simulink model "blocks_archive"  (R2019b)
settings: Solver=VariableStepAuto  StartTime=0.0  StopTime=10.0  RelTol=1e-3
values from neighbouring files (symbols this model uses):
  a = input("Semimajor axis [km]: ")    [SCARSSetup.m]    (also in pwsat2_setup.m = 6960989.91401; pwsat2_tle.m = 6960989.91401; scars_setup.m = 8000000; startup.m = 8000000)
  e = input("Eccentricity [-]: ")    [SCARSSetup.m]    (also in pwsat2_setup.m = 0.0011871; pwsat2_tle.m = 0.0011871; scars_setup.m = 0; startup.m = 0)
  G = 6.6743015e-11    [SCARSSetup.m]    (also in pwsat2_setup.m; pwsat2_tle.m; scars_setup.m; startup.m)
  h = norm(H)    [eci2kep.m]    (also in kep2eci.m = sqrt(a*mu*(1-e^2)); kep2rv.m = sqrt(a*mu*(1-e^2)); pwsat2_setup.m = 6378000; pwsat2_tle.m = 6378000)
  incl = input("Inclination [deg]: ")    [SCARSSetup.m]    (also in pwsat2_setup.m = deg2rad(97.7672); pwsat2_tle.m = deg2rad(97.7672); scars_setup.m = deg2rad(0.00000001); startup.m = deg2rad(45))
  Me = 5.972e24    (= 5.972e+24)    [SCARSSetup.m]    (also in pwsat2_setup.m; pwsat2_tle.m; scars_setup.m; startup.m)
  mu = 398600.4418    [eci2kep.m]    (also in pwsat2_setup.m = 398600441800000; pwsat2_tle.m = 398600441800000; scars_setup.m = 398600441800000; startup.m = 398600441800000)
  omega = 7.2921150e-5    (= 7.292115e-05)    [SCARSSetup.m]    (also in ec2ecef_test.m; pwsat2_setup.m; pwsat2_tle.m; scars_setup.m)
  RA = input("Right ascension of the ascending node [deg]: ")    [SCARSSetup.m]    (also in pwsat2_setup.m = deg2rad(56.1804); pwsat2_tle.m = deg2rad(56.1804); scars_setup.m = deg2rad(180); startup.m = deg2rad(90))
  TA = deg2rad(0)    [scars_setup.m]    (also in startup.m; startup_cubesat_ref.m = deg2rad(302.9234))
  v0 = [0 vy 0]    [startup.m]    (also in startup_cubesat_ref.m)
  w = input("Argument of periapsis [deg]: ")    [SCARSSetup.m]    (also in pwsat2_setup.m = deg2rad(236.0402); pwsat2_tle.m = deg2rad(236.0402); scars_setup.m = deg2rad(0); startup.m = deg2rad(0))
undefined symbols (not defined in the file or in its folder): IAU
libraries: sharedutil x6, aerolibgravity2 x2, aerolibtransform2 x1
settings Model: Creator=asmialek  LastModifiedBy=asmialek

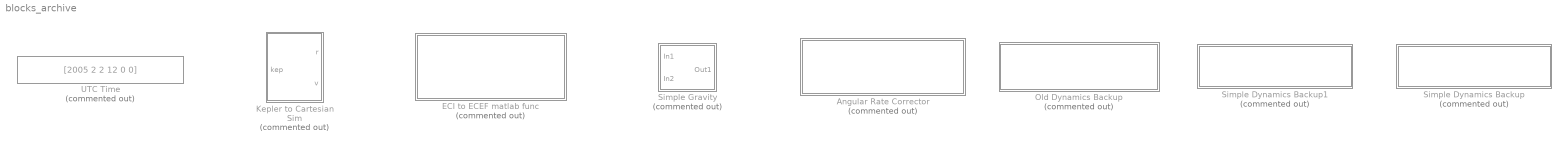
== system blocks_archive ==
  Angular Rate Corrector : Subsystem  Commented=on
  ECI to ECEF matlab func : Subsystem  Commented=on
  Kepler to Cartesian Sim : Subsystem  Commented=on
  Old Dynamics Backup : Subsystem  Commented=on
  Simple Dynamics Backup : Subsystem  Commented=on
  Simple Dynamics Backup1 : Subsystem  Commented=on
  Simple Gravity : Subsystem  Commented=on
  UTC Time : Constant  Commented=on  Value=[2005 2 2 12 0 0]

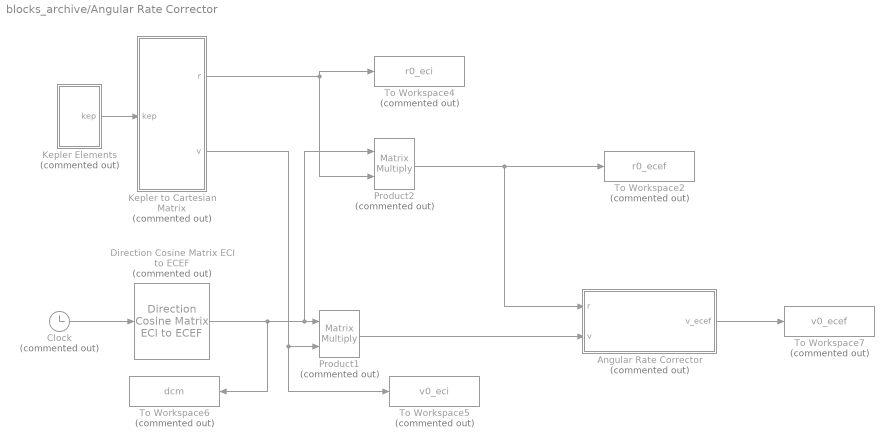
== system blocks_archive/Angular Rate Corrector ==
  Angular Rate Corrector : Subsystem  Commented=on
  Clock : Clock  Commented=on
  Direction Cosine Matrix ECI to ECEF : aerolibtransform2/Direction Cosine Matrix ECI to ECEF  Commented=on  red=IAU-2000/2006  year=2005  month=February  day=2  hour=12  min=0  sec=0  deltaT=Sec  errorflag=Error  extraparamflag=off
      settings: AttributesFormatString=%<red>  SourceProductName=Aerospace Blockset  SourceProductBaseCode=AE
  Kepler Elements : Subsystem  Commented=on
  Kepler to Cartesian Matrix : Subsystem  Commented=on
  Product1 : Product  Commented=on  Multiplication=Matrix(*)
  Product2 : Product  Commented=on  Multiplication=Matrix(*)
  To Workspace2 : ToWorkspace  Commented=on  VariableName=r0_ecef  SampleTime=-1
  To Workspace4 : ToWorkspace  Commented=on  VariableName=r0_eci  SampleTime=-1
  To Workspace5 : ToWorkspace  Commented=on  VariableName=v0_eci  SampleTime=-1
  To Workspace6 : ToWorkspace  Commented=on  VariableName=dcm  SampleTime=-1
  To Workspace7 : ToWorkspace  Commented=on  VariableName=v0_ecef  SampleTime=-1
  wires:
  Kepler to Cartesian Matrix/1(r) -> To Workspace4/1, Product2/2
  Direction Cosine Matrix ECI to ECEF/1 -> To Workspace6/1, Product2/1, Product1/1
  Clock/1 -> Direction Cosine Matrix ECI to ECEF/1
  Product1/1 -> Angular Rate Corrector/2(v)
  Product2/1 -> To Workspace2/1, Angular Rate Corrector/1(r)
  Kepler to Cartesian Matrix/2(v) -> To Workspace5/1, Product1/2
  Angular Rate Corrector/1(v_ecef) -> To Workspace7/1
  Kepler Elements/1(kep) -> Kepler to Cartesian Matrix/1(kep)

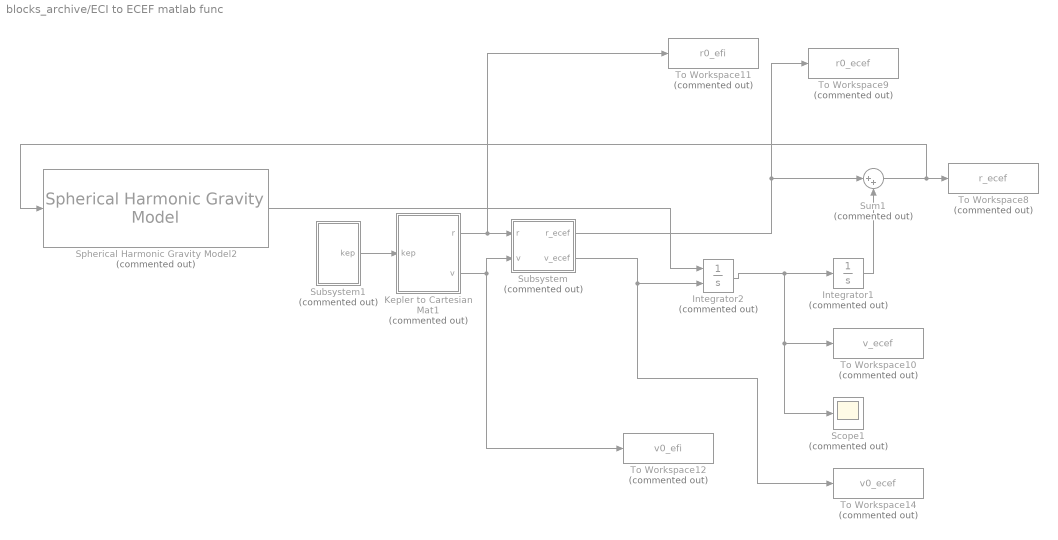
== system blocks_archive/ECI to ECEF matlab func ==
  Integrator1 : Integrator  Commented=on
  Integrator2 : Integrator  Commented=on  InitialConditionSource=external
  Kepler to Cartesian Mat1 : Subsystem  Commented=on
  Scope1 : Scope  Commented=on
  Spherical Harmonic Gravity Model2 : aerolibgravity2/Spherical Harmonic Gravity Model  Commented=on  units=Metric (MKS)  degree=120  action=Warning  ptype=EGM2008  datafile='aerogmm2b.mat'
      settings: SourceProductName=Aerospace Blockset  SourceProductBaseCode=AE
  Subsystem : Subsystem  Commented=on
  Subsystem1 : Subsystem  Commented=on
  Sum1 : Sum  Commented=on  Inputs=|++
  To Workspace10 : ToWorkspace  Commented=on  VariableName=v_ecef  SampleTime=-1
      settings: Save2DSignal=2-D array (concatenate along first dimension)
  To Workspace11 : ToWorkspace  Commented=on  VariableName=r0_efi  SampleTime=-1
  To Workspace12 : ToWorkspace  Commented=on  VariableName=v0_efi  SampleTime=-1
  To Workspace14 : ToWorkspace  Commented=on  VariableName=v0_ecef  SampleTime=-1
  To Workspace8 : ToWorkspace  Commented=on  VariableName=r_ecef  SampleTime=-1
  To Workspace9 : ToWorkspace  Commented=on  VariableName=r0_ecef  SampleTime=-1
  wires:
  Integrator2/1 -> Scope1/1, To Workspace10/1, Integrator1/1
  Sum1/1 -> To Workspace8/1, Spherical Harmonic Gravity Model2/1
  Kepler to Cartesian Mat1/2(v) -> Subsystem/2(v), To Workspace12/1
  Spherical Harmonic Gravity Model2/1 -> Integrator2/1
  Subsystem/1(r_ecef) -> To Workspace9/1, Sum1/1
  Integrator1/1 -> Sum1/2
  Subsystem1/1(kep) -> Kepler to Cartesian Mat1/1(kep)
  Kepler to Cartesian Mat1/1(r) -> To Workspace11/1, Subsystem/1(r)
  Subsystem/2(v_ecef) -> To Workspace14/1, Integrator2/2

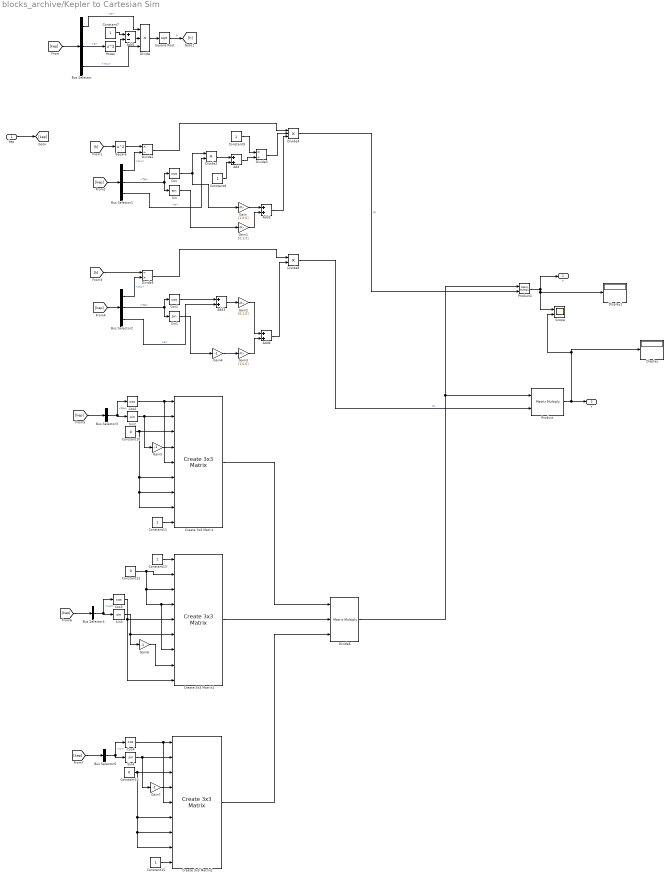
== system blocks_archive/Kepler to Cartesian Sim ==
  kep : Inport
  Add{,2..4} (4 alike) : Sum
  Add1 : Sum  Inputs=+-
  Bus Selector : BusSelector  OutputSignals=a,e,mu
  Bus Selector1 : BusSelector  OutputSignals=mu,TA,e
  Bus Selector2 : BusSelector  OutputSignals=mu,TA,e
  Bus Selector3 : BusSelector  OutputSignals=RA
  Bus Selector4 : BusSelector  OutputSignals=incl
  Bus Selector5 : BusSelector  OutputSignals=w
  Constant10 : Constant  Value=0
  Constant{7..9,11,13,15} (6 alike) : Constant
  Constant12 : Constant  Value=0
  Constant14 : Constant  Value=0
  Cos{,1..4} (5 alike) : Trigonometry  Operator=cos
  Create 3x3 Matrix : sharedutil/Create 3x3 Matrix  aMode=aMode
  Create 3x3 Matrix1 : sharedutil/Create 3x3 Matrix  aMode=aMode
  Create 3x3 Matrix2 : sharedutil/Create 3x3 Matrix  aMode=aMode
  Display : Display
  Display1 : Display
  Divide : Product  Inputs=3
  Divide1 : Product  Inputs=*/
  Divide2 : Product
  Divide3 : Product  Inputs=*/
  Divide4 : Product  Inputs=3
  Divide5 : Product  Inputs=/*
  Divide6 : Product  Inputs=3  Multiplication=Matrix(*)
  Divide8 : Product
  Gain : Gain  Gain=[1;0;0]
  Gain1 : Gain  Gain=[0;1;0]
  Gain2 : Gain  Gain=[0;1;0]
  Gain3 : Gain  Gain=[1;0;0]
  Gain{4..7} (4 alike) : Gain  Gain=-1
  Power : Math  Operator=square  SignedPower=off  SaturateOnIntegerOverflow=on
  Product : Product  Multiplication=Matrix(*)
  Product1 : Product  Multiplication=Matrix(*)
  Scope : Scope  NumInputPorts=2
  Sin{,1..4} (5 alike) : Trigonometry
  Square : Math  Operator=square  SignedPower=off  SaturateOnIntegerOverflow=on
  Square Root : Sqrt  SaturateOnIntegerOverflow=on
  r : Outport
  v : Outport  Port=2
  wires:
  Bus Selector2/1 -> Divide5/2  "<mu>"
  [h] -> Square/1
  Square Root/1 -> [h]  "h"
  Bus Selector2/3 -> Add3/2  "<e>"
  [kep] -> Bus Selector3/1
  Gain5/1 -> Create 3x3 Matrix/4
  Divide3/1 -> Divide4/2
  Constant15/1 -> Create 3x3 Matrix2/9
  Bus Selector1/1 -> Divide1/2  "<mu>"
  Gain6/1 -> Create 3x3 Matrix1/8
  Add/1 -> Divide3/2
  Create 3x3 Matrix2/1 -> Divide6/3
  Divide1/1 -> Divide4/1
  Sin1/1 -> Gain4/1
  Cos1/1 -> Add3/1
  Gain7/1 -> Create 3x3 Matrix2/4
  Gain3/1 -> Add4/2
  Cos2/1 -> Create 3x3 Matrix/5, Create 3x3 Matrix/1
  [kep] -> Bus Selector4/1
  Gain1/1 -> Add2/2
  Constant7/1 -> Add1/1
  Create 3x3 Matrix1/1 -> Divide6/2
  Divide5/1 -> Divide8/1
  Bus Selector4/1 -> Cos3/1, Sin3/1  "<incl>"
  Constant10/1 -> Create 3x3 Matrix/8, Create 3x3 Matrix/7, Create 3x3 Matrix/6, Create 3x3 Matrix/3
  Divide6/1 -> Product1/1, Product/1
  Cos3/1 -> Create 3x3 Matrix1/9, Create 3x3 Matrix1/5
  Power/1 -> Add1/2
  [kep] -> Bus Selector/1
  Constant12/1 -> Create 3x3 Matrix1/7, Create 3x3 Matrix1/4, Create 3x3 Matrix1/3, Create 3x3 Matrix1/2
  Bus Selector1/2 -> Cos/1, Sin/1  "<TA>"
  Bus Selector/3 -> Divide/3  "<mu>"
  Divide4/1 -> Product1/2  "rp"
  Bus Selector5/1 -> Cos4/1, Sin4/1  "<w>"
  Gain2/1 -> Add4/1
  Sin4/1 -> Gain7/1, Create 3x3 Matrix2/2
  Bus Selector1/3 -> Divide2/2  "<e>"
  [kep] -> Bus Selector5/1
  Gain4/1 -> Gain3/1
  Divide2/1 -> Add/1
  kep/1 -> [kep]
  [kep] -> Bus Selector1/1
  Sin3/1 -> Create 3x3 Matrix1/6, Gain6/1
  Divide8/1 -> Product/2  "vp"
  Constant13/1 -> Create 3x3 Matrix1/1
  [kep] -> Bus Selector2/1
  Bus Selector3/1 -> Cos2/1, Sin2/1  "<RA>"
  Constant8/1 -> Add/2
  Add4/1 -> Divide8/2
  Bus Selector/1 -> Divide/1  "<a>"
  Sin/1 -> Gain1/1
  Product1/1 -> r/1, Display1/1, Scope/1
  Bus Selector2/2 -> Cos1/1, Sin1/1  "<TA>"
  Add2/1 -> Divide4/3
  Add3/1 -> Gain2/1
  Constant11/1 -> Create 3x3 Matrix/9
  Constant14/1 -> Create 3x3 Matrix2/8, Create 3x3 Matrix2/7, Create 3x3 Matrix2/6, Create 3x3 Matrix2/3
  Create 3x3 Matrix/1 -> Divide6/1
  Product/1 -> v/1, Display/1, Scope/2
  Add1/1 -> Divide/2
  [h] -> Divide5/1
  Divide/1 -> Square Root/1
  Bus Selector/2 -> Power/1  "<e>"
  Cos4/1 -> Create 3x3 Matrix2/5, Create 3x3 Matrix2/1
  Sin2/1 -> Gain5/1, Create 3x3 Matrix/2
  Square/1 -> Divide1/1
  Cos/1 -> Divide2/1, Gain/1
  Constant9/1 -> Divide3/1
  Gain/1 -> Add2/1

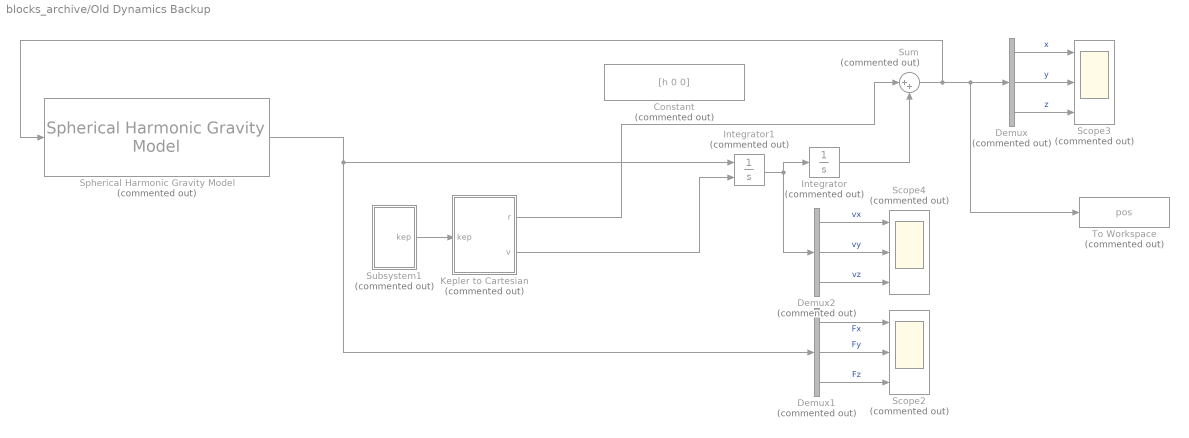
== system blocks_archive/Old Dynamics Backup ==
  Constant : Constant  Commented=on  Value=[h 0 0]
  Demux : Demux  Commented=on  Outputs=3
  Demux1 : Demux  Commented=on  Outputs=3
  Demux2 : Demux  Commented=on  Outputs=3
  Integrator : Integrator  Commented=on
  Integrator1 : Integrator  Commented=on  InitialConditionSource=external  InitialCondition=v0
  Kepler to Cartesian : Subsystem  Commented=on
  Scope2 : Scope  Commented=on  NumInputPorts=3
  Scope3 : Scope  Commented=on  NumInputPorts=3
  Scope4 : Scope  Commented=on  NumInputPorts=3
  Spherical Harmonic Gravity Model : aerolibgravity2/Spherical Harmonic Gravity Model  Commented=on  units=Metric (MKS)  degree=120  action=Warning  ptype=EGM2008  datafile='aerogmm2b.mat'
      settings: SourceProductName=Aerospace Blockset  SourceProductBaseCode=AE
  Subsystem1 : Subsystem  Commented=on
  Sum : Sum  Commented=on  Inputs=|++
  To Workspace : ToWorkspace  Commented=on  VariableName=pos  SampleTime=-1
  wires:
  Demux/1 -> Scope3/1  "x"
  Demux/3 -> Scope3/3  "z"
  Subsystem1/1(kep) -> Kepler to Cartesian/1(kep)
  Demux1/1 -> Scope2/1  "Fx"
  Kepler to Cartesian/2(v) -> Integrator1/2
  Demux1/2 -> Scope2/2  "Fy"
  Integrator1/1 -> Integrator/1, Demux2/1
  Demux1/3 -> Scope2/3  "Fz"
  Spherical Harmonic Gravity Model/1 -> Integrator1/1, Demux1/1
  Demux2/3 -> Scope4/3  "vz"
  Sum/1 -> To Workspace/1, Demux/1, Spherical Harmonic Gravity Model/1
  Kepler to Cartesian/1(r) -> Sum/1
  Demux2/2 -> Scope4/2  "vy"
  Integrator/1 -> Sum/2
  Demux/2 -> Scope3/2  "y"
  Demux2/1 -> Scope4/1  "vx"

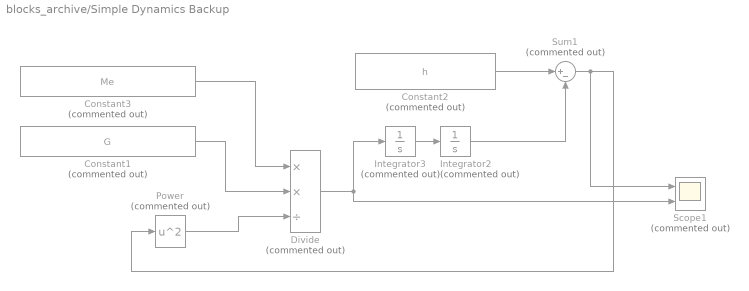
== system blocks_archive/Simple Dynamics Backup ==
  Constant1 : Constant  Commented=on  Value=G
  Constant2 : Constant  Commented=on  Value=h
  Constant3 : Constant  Commented=on  Value=Me
  Divide : Product  Commented=on  Inputs=**/
  Integrator2 : Integrator  Commented=on
  Integrator3 : Integrator  Commented=on
  Power : Math  Commented=on  Operator=square  SignedPower=off  SaturateOnIntegerOverflow=on
  Scope1 : Scope  Commented=on  NumInputPorts=2
  Sum1 : Sum  Commented=on  Inputs=|+-
  wires:
  Constant2/1 -> Sum1/1
  Constant1/1 -> Divide/2
  Integrator3/1 -> Integrator2/1
  Constant3/1 -> Divide/1
  Power/1 -> Divide/3
  Divide/1 -> Integrator3/1, Scope1/2
  Integrator2/1 -> Sum1/2
  Sum1/1 -> Scope1/1, Power/1

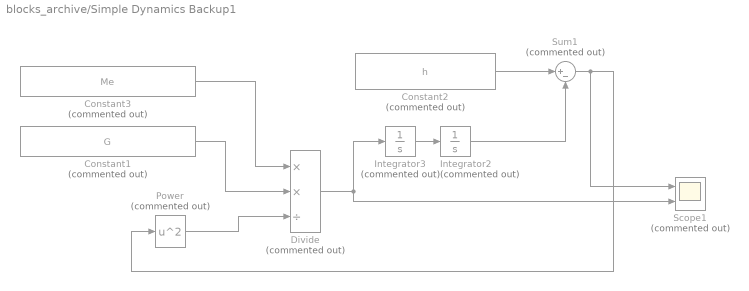
== system blocks_archive/Simple Dynamics Backup1 ==
  Constant1 : Constant  Commented=on  Value=G
  Constant2 : Constant  Commented=on  Value=h
  Constant3 : Constant  Commented=on  Value=Me
  Divide : Product  Commented=on  Inputs=**/
  Integrator2 : Integrator  Commented=on
  Integrator3 : Integrator  Commented=on
  Power : Math  Commented=on  Operator=square  SignedPower=off  SaturateOnIntegerOverflow=on
  Scope1 : Scope  Commented=on  NumInputPorts=2
  Sum1 : Sum  Commented=on  Inputs=|+-
  wires:
  Constant2/1 -> Sum1/1
  Constant1/1 -> Divide/2
  Integrator3/1 -> Integrator2/1
  Constant3/1 -> Divide/1
  Power/1 -> Divide/3
  Divide/1 -> Integrator3/1, Scope1/2
  Integrator2/1 -> Sum1/2
  Sum1/1 -> Scope1/1, Power/1

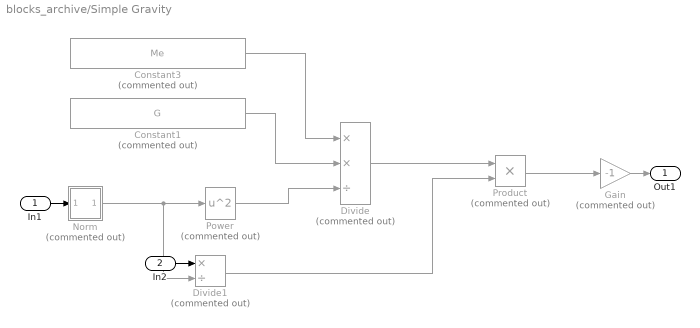
== system blocks_archive/Simple Gravity ==
  In1 : Inport
  In2 : Inport  Port=2
  Constant1 : Constant  Commented=on  Value=G
  Constant3 : Constant  Commented=on  Value=Me
  Divide : Product  Commented=on  Inputs=**/
  Divide1 : Product  Commented=on  Inputs=*/
  Gain : Gain  Commented=on  Gain=-1
  Norm : Subsystem  Commented=on
  Power : Math  Commented=on  Operator=square  SignedPower=off  SaturateOnIntegerOverflow=on
  Product : Product  Commented=on
  Out1 : Outport
  wires:
  Divide/1 -> Product/1
  Power/1 -> Divide/3
  Constant1/1 -> Divide/2
  In1/1 -> Norm/1(In1)
  Divide1/1 -> Product/2
  Norm/1(Out1) -> Divide1/2, Power/1
  Product/1 -> Gain/1
  Constant3/1 -> Divide/1
  Gain/1 -> Out1/1
  In2/1 -> Divide1/1

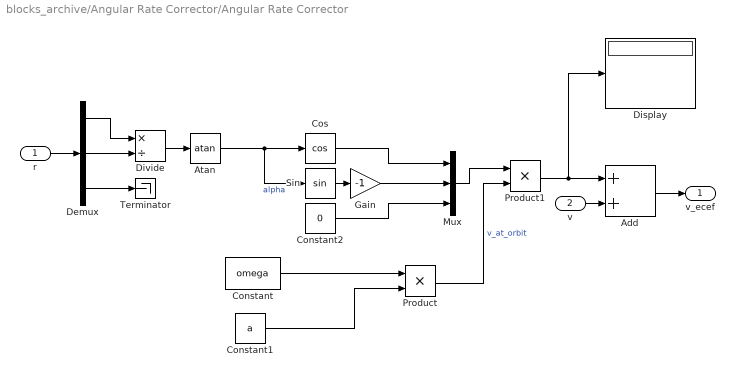
== system blocks_archive/Angular Rate Corrector/Angular Rate Corrector ==
  r : Inport
  v : Inport  Port=2
  Add : Sum
  Atan : Trigonometry  Operator=atan
  Constant : Constant  Value=omega
  Constant1 : Constant  Value=a
  Constant2 : Constant  Value=0
  Cos : Trigonometry  Operator=cos
  Demux : Demux  Outputs=3
  Display : Display
  Divide : Product  Inputs=*/
  Gain : Gain  Gain=-1
  Mux : Mux  Inputs=3
  Product : Product
  Product1 : Product
  Sin : Trigonometry
  Terminator : Terminator
  v_ecef : Outport
  wires:
  Add/1 -> v_ecef/1
  Product1/1 -> Display/1, Add/1
  r/1 -> Demux/1
  Demux/1 -> Divide/1
  Demux/2 -> Divide/2
  Divide/1 -> Atan/1
  Demux/3 -> Terminator/1
  Atan/1 -> Sin/1, Cos/1  "alpha"
  Constant/1 -> Product/1
  Constant1/1 -> Product/2
  Product/1 -> Product1/2  "v_at_orbit"
  v/1 -> Add/2
  Constant2/1 -> Mux/3
  Cos/1 -> Mux/1
  Sin/1 -> Gain/1
  Gain/1 -> Mux/2
  Mux/1 -> Product1/1

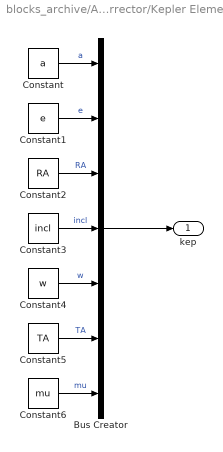
== system blocks_archive/Angular Rate Corrector/Kepler Elements ==
  Bus Creator : BusCreator  Inputs=7
  Constant : Constant  Value=a
  Constant1 : Constant  Value=e
  Constant2 : Constant  Value=RA
  Constant3 : Constant  Value=incl
  Constant4 : Constant  Value=w
  Constant5 : Constant  Value=TA
  Constant6 : Constant  Value=mu
  kep : Outport
  wires:
  Constant4/1 -> Bus Creator/5  "w"
  Constant/1 -> Bus Creator/1  "a"
  Bus Creator/1 -> kep/1
  Constant2/1 -> Bus Creator/3  "RA"
  Constant1/1 -> Bus Creator/2  "e"
  Constant3/1 -> Bus Creator/4  "incl"
  Constant5/1 -> Bus Creator/6  "TA"
  Constant6/1 -> Bus Creator/7  "mu"

== system blocks_archive/Angular Rate Corrector/Kepler to Cartesian Matrix ==
  kep : Inport
  Bus Selector : BusSelector  OutputSignals=a,e,RA,incl,w,TA,mu
  MATLAB Function : MATLAB Function  TreatAsAtomicUnit=on
  r : Outport
  v : Outport  Port=2
  wires:
  kep/1 -> Bus Selector/1
  Bus Selector/1 -> MATLAB Function/1(a)  "<a>"
  Bus Selector/2 -> MATLAB Function/2(e)  "<e>"
  Bus Selector/4 -> MATLAB Function/4(incl)  "<incl>"
  Bus Selector/5 -> MATLAB Function/5(w)  "<w>"
  Bus Selector/6 -> MATLAB Function/6(TA)  "<TA>"
  Bus Selector/7 -> MATLAB Function/7(mu)  "<mu>"
  Bus Selector/3 -> MATLAB Function/3(RA)  "<RA>"
  MATLAB Function/1(r) -> r/1
  MATLAB Function/2(v) -> v/1

== system blocks_archive/ECI to ECEF matlab func/Kepler to Cartesian Mat1 ==
  kep : Inport
  Bus Selector : BusSelector  OutputSignals=a,e,RA,incl,w,TA,mu
  MATLAB Function : MATLAB Function  TreatAsAtomicUnit=on
  r : Outport
  v : Outport  Port=2
  wires:
  kep/1 -> Bus Selector/1
  Bus Selector/1 -> MATLAB Function/1(a)  "<a>"
  Bus Selector/2 -> MATLAB Function/2(e)  "<e>"
  Bus Selector/4 -> MATLAB Function/4(incl)  "<incl>"
  Bus Selector/5 -> MATLAB Function/5(w)  "<w>"
  Bus Selector/6 -> MATLAB Function/6(TA)  "<TA>"
  Bus Selector/7 -> MATLAB Function/7(mu)  "<mu>"
  Bus Selector/3 -> MATLAB Function/3(RA)  "<RA>"
  MATLAB Function/1(r) -> r/1
  MATLAB Function/2(v) -> v/1

== system blocks_archive/ECI to ECEF matlab func/Subsystem ==
  r : Inport
  v : Inport  Port=2
  Constant : Constant  Value=[0 0 0]
  Constant1 : Constant  Value=2453404
  MATLAB Function : MATLAB Function  TreatAsAtomicUnit=on
  Terminator : Terminator
  r_ecef : Outport
  v_ecef : Outport  Port=2
  wires:
  Constant/1 -> MATLAB Function/4(a_ECI)
  v/1 -> MATLAB Function/3(v_ECI)
  MATLAB Function/2(v_ECEF) -> v_ecef/1
  MATLAB Function/3(a_ECEF) -> Terminator/1
  Constant1/1 -> MATLAB Function/1(JD)
  MATLAB Function/1(r_ECEF) -> r_ecef/1
  r/1 -> MATLAB Function/2(r_ECI)

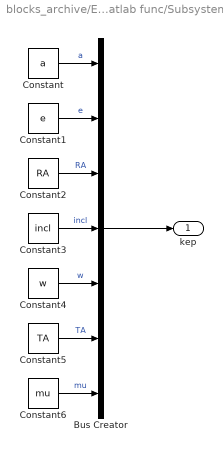
== system blocks_archive/ECI to ECEF matlab func/Subsystem1 ==
  Bus Creator : BusCreator  Inputs=7
  Constant : Constant  Value=a
  Constant1 : Constant  Value=e
  Constant2 : Constant  Value=RA
  Constant3 : Constant  Value=incl
  Constant4 : Constant  Value=w
  Constant5 : Constant  Value=TA
  Constant6 : Constant  Value=mu
  kep : Outport
  wires:
  Constant4/1 -> Bus Creator/5  "w"
  Constant/1 -> Bus Creator/1  "a"
  Bus Creator/1 -> kep/1
  Constant2/1 -> Bus Creator/3  "RA"
  Constant1/1 -> Bus Creator/2  "e"
  Constant3/1 -> Bus Creator/4  "incl"
  Constant5/1 -> Bus Creator/6  "TA"
  Constant6/1 -> Bus Creator/7  "mu"

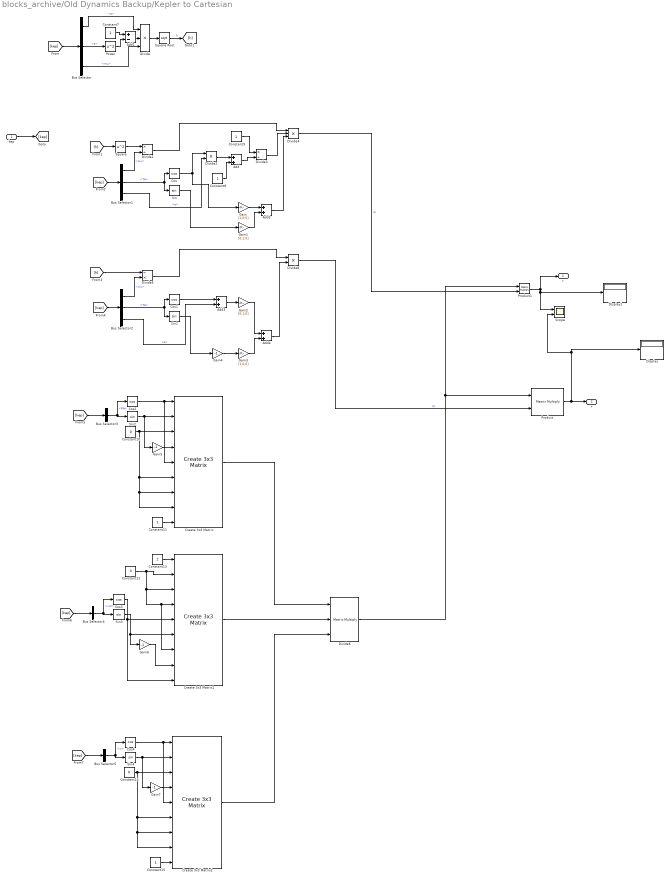
== system blocks_archive/Old Dynamics Backup/Kepler to Cartesian ==
  kep : Inport
  Add{,2..4} (4 alike) : Sum
  Add1 : Sum  Inputs=+-
  Bus Selector : BusSelector  OutputSignals=a,e,mu
  Bus Selector1 : BusSelector  OutputSignals=mu,TA,e
  Bus Selector2 : BusSelector  OutputSignals=mu,TA,e
  Bus Selector3 : BusSelector  OutputSignals=RA
  Bus Selector4 : BusSelector  OutputSignals=incl
  Bus Selector5 : BusSelector  OutputSignals=w
  Constant10 : Constant  Value=0
  Constant{7..9,11,13,15} (6 alike) : Constant
  Constant12 : Constant  Value=0
  Constant14 : Constant  Value=0
  Cos{,1..4} (5 alike) : Trigonometry  Operator=cos
  Create 3x3 Matrix : sharedutil/Create 3x3 Matrix  aMode=aMode
  Create 3x3 Matrix1 : sharedutil/Create 3x3 Matrix  aMode=aMode
  Create 3x3 Matrix2 : sharedutil/Create 3x3 Matrix  aMode=aMode
  Display : Display
  Display1 : Display
  Divide : Product  Inputs=3
  Divide1 : Product  Inputs=*/
  Divide2 : Product
  Divide3 : Product  Inputs=*/
  Divide4 : Product  Inputs=3
  Divide5 : Product  Inputs=/*
  Divide6 : Product  Inputs=3  Multiplication=Matrix(*)
  Divide8 : Product
  Gain : Gain  Gain=[1;0;0]
  Gain1 : Gain  Gain=[0;1;0]
  Gain2 : Gain  Gain=[0;1;0]
  Gain3 : Gain  Gain=[1;0;0]
  Gain{4..7} (4 alike) : Gain  Gain=-1
  Power : Math  Operator=square  SignedPower=off  SaturateOnIntegerOverflow=on
  Product : Product  Multiplication=Matrix(*)
  Product1 : Product  Multiplication=Matrix(*)
  Scope : Scope  NumInputPorts=2
  Sin{,1..4} (5 alike) : Trigonometry
  Square : Math  Operator=square  SignedPower=off  SaturateOnIntegerOverflow=on
  Square Root : Sqrt  SaturateOnIntegerOverflow=on
  r : Outport
  v : Outport  Port=2
  wires:
  Bus Selector2/1 -> Divide5/2  "<mu>"
  [h] -> Square/1
  Square Root/1 -> [h]  "h"
  Bus Selector2/3 -> Add3/2  "<e>"
  [kep] -> Bus Selector3/1
  Gain5/1 -> Create 3x3 Matrix/4
  Divide3/1 -> Divide4/2
  Constant15/1 -> Create 3x3 Matrix2/9
  Bus Selector1/1 -> Divide1/2  "<mu>"
  Gain6/1 -> Create 3x3 Matrix1/8
  Add/1 -> Divide3/2
  Create 3x3 Matrix2/1 -> Divide6/3
  Divide1/1 -> Divide4/1
  Sin1/1 -> Gain4/1
  Cos1/1 -> Add3/1
  Gain7/1 -> Create 3x3 Matrix2/4
  Gain3/1 -> Add4/2
  Cos2/1 -> Create 3x3 Matrix/5, Create 3x3 Matrix/1
  [kep] -> Bus Selector4/1
  Gain1/1 -> Add2/2
  Constant7/1 -> Add1/1
  Create 3x3 Matrix1/1 -> Divide6/2
  Divide5/1 -> Divide8/1
  Bus Selector4/1 -> Cos3/1, Sin3/1  "<incl>"
  Constant10/1 -> Create 3x3 Matrix/8, Create 3x3 Matrix/7, Create 3x3 Matrix/6, Create 3x3 Matrix/3
  Divide6/1 -> Product1/1, Product/1
  Cos3/1 -> Create 3x3 Matrix1/9, Create 3x3 Matrix1/5
  Power/1 -> Add1/2
  [kep] -> Bus Selector/1
  Constant12/1 -> Create 3x3 Matrix1/7, Create 3x3 Matrix1/4, Create 3x3 Matrix1/3, Create 3x3 Matrix1/2
  Bus Selector1/2 -> Cos/1, Sin/1  "<TA>"
  Bus Selector/3 -> Divide/3  "<mu>"
  Divide4/1 -> Product1/2  "rp"
  Bus Selector5/1 -> Cos4/1, Sin4/1  "<w>"
  Gain2/1 -> Add4/1
  Sin4/1 -> Gain7/1, Create 3x3 Matrix2/2
  Bus Selector1/3 -> Divide2/2  "<e>"
  [kep] -> Bus Selector5/1
  Gain4/1 -> Gain3/1
  Divide2/1 -> Add/1
  kep/1 -> [kep]
  [kep] -> Bus Selector1/1
  Sin3/1 -> Create 3x3 Matrix1/6, Gain6/1
  Divide8/1 -> Product/2  "vp"
  Constant13/1 -> Create 3x3 Matrix1/1
  [kep] -> Bus Selector2/1
  Bus Selector3/1 -> Cos2/1, Sin2/1  "<RA>"
  Constant8/1 -> Add/2
  Add4/1 -> Divide8/2
  Bus Selector/1 -> Divide/1  "<a>"
  Sin/1 -> Gain1/1
  Product1/1 -> r/1, Display1/1, Scope/1
  Bus Selector2/2 -> Cos1/1, Sin1/1  "<TA>"
  Add2/1 -> Divide4/3
  Add3/1 -> Gain2/1
  Constant11/1 -> Create 3x3 Matrix/9
  Constant14/1 -> Create 3x3 Matrix2/8, Create 3x3 Matrix2/7, Create 3x3 Matrix2/6, Create 3x3 Matrix2/3
  Create 3x3 Matrix/1 -> Divide6/1
  Product/1 -> v/1, Display/1, Scope/2
  Add1/1 -> Divide/2
  [h] -> Divide5/1
  Divide/1 -> Square Root/1
  Bus Selector/2 -> Power/1  "<e>"
  Cos4/1 -> Create 3x3 Matrix2/5, Create 3x3 Matrix2/1
  Sin2/1 -> Gain5/1, Create 3x3 Matrix/2
  Square/1 -> Divide1/1
  Cos/1 -> Divide2/1, Gain/1
  Constant9/1 -> Divide3/1
  Gain/1 -> Add2/1

== system blocks_archive/Old Dynamics Backup/Subsystem1 ==
  Bus Creator : BusCreator  Inputs=7
  Constant : Constant  Value=a
  Constant1 : Constant  Value=e
  Constant2 : Constant  Value=RA
  Constant3 : Constant  Value=incl
  Constant4 : Constant  Value=w
  Constant5 : Constant  Value=TA
  Constant6 : Constant  Value=mu
  kep : Outport
  wires:
  Constant4/1 -> Bus Creator/5  "w"
  Constant/1 -> Bus Creator/1  "a"
  Bus Creator/1 -> kep/1
  Constant2/1 -> Bus Creator/3  "RA"
  Constant1/1 -> Bus Creator/2  "e"
  Constant3/1 -> Bus Creator/4  "incl"
  Constant5/1 -> Bus Creator/6  "TA"
  Constant6/1 -> Bus Creator/7  "mu"

== system blocks_archive/Simple Gravity/Norm ==
  In1 : Inport
  Dot Product : DotProduct  InputSameDT=on  OutDataTypeStr=Inherit: Inherit via internal rule
  Square Root : Sqrt  SaturateOnIntegerOverflow=on
  Out1 : Outport
  wires:
  Dot Product/1 -> Square Root/1
  In1/1 -> Dot Product/2, Dot Product/1
  Square Root/1 -> Out1/1

== matlab function blocks_archive/ECI to ECEF matlab func/Kepler to Cartesian Mat1/MATLAB Function ==
  data: a input; r output; e input; RA input; incl input; w input; TA input; mu input; v output
% h - angular momentum (km^2/s)
% e - eccentricity (unitless)
% RA - right ascension of the ascending node (rad)
% incl - inclination (rad)
% w - argument of periapis (rad)
% TA - true anomaly (rad)
% mu - standard gravitational parameter (m^3/s^2)

function [r, v] = kep2rv(a, e, RA, incl, w, TA, mu)

h = sqrt(a*mu*(1-e^2));

rp = (h^2/mu) * (1/(1 + e.*cos(TA))) * (cos(TA).*[1;0;0] + sin(TA).*[0;1;0]);
vp = (mu/h) * (-sin(TA).*[1;0;0] + (e + cos(TA)).*[0;1;0]);

R3_W = [ cos(RA) sin(RA) 0;
         -sin(RA) cos(RA) 0;
         0          0       1];
     
R1_i = [1 0 0;
        0 cos(incl) sin(incl);
        0 -sin(incl) cos(incl)];
    
R3_w = [ cos(w) sin(w) 0;
         -sin(w) cos(w) 0;
         0 0 1];
     
Q_pX = (R3_w*R1_i*R3_W)';

r = Q_pX*rp;
v = Q_pX*vp;

r = r;
v = v;

end

== matlab function blocks_archive/Angular Rate Corrector/Kepler to Cartesian Matrix/MATLAB Function ==
  data: a input; r output; e input; RA input; incl input; w input; TA input; mu input; v output
% h - angular momentum (km^2/s)
% e - eccentricity (unitless)
% RA - right ascension of the ascending node (rad)
% incl - inclination (rad)
% w - argument of periapis (rad)
% TA - true anomaly (rad)
% mu - standard gravitational parameter (m^3/s^2)

function [r, v] = kep2rv(a, e, RA, incl, w, TA, mu)

h = sqrt(a*mu*(1-e^2));

rp = (h^2/mu) * (1/(1 + e.*cos(TA))) * (cos(TA).*[1;0;0] + sin(TA).*[0;1;0]);
vp = (mu/h) * (-sin(TA).*[1;0;0] + (e + cos(TA)).*[0;1;0]);

R3_W = [ cos(RA) sin(RA) 0;
         -sin(RA) cos(RA) 0;
         0          0       1];
     
R1_i = [1 0 0;
        0 cos(incl) sin(incl);
        0 -sin(incl) cos(incl)];
    
R3_w = [ cos(w) sin(w) 0;
         -sin(w) cos(w) 0;
         0 0 1];
     
Q_pX = (R3_w*R1_i*R3_W)';

r = Q_pX*rp;
v = Q_pX*vp;

r = r;
v = v;

end

== matlab function blocks_archive/ECI to ECEF matlab func/Subsystem/MATLAB Function ==
  data: JD input; r_ECEF output; r_ECI input; v_ECI input; a_ECI input; v_ECEF output; a_ECEF output
%----------------------- Begin Code Sequence -----------------------------%
% Purpose:                                                                %
% Convert ECI (CIS, Epoch J2000.0) Coordinates to WGS 84 (CTS, ECEF)      %
% Coordinates. This function has been vectorized for speed.               %
%                                                                         %
% Inputs:                                                                 %
%-------                                                                  %
%JD                     [1 x N]                         Julian Date Vector
%
%r_ECI                  [3 x N]                         Position Vector
%                                                       in ECI coordinate
%                                                       frame of reference
%
%v_ECI                  [3 x N]                         Velocity Vector in
%                                                       ECI coordinate
%                                                       frame of reference
%
%a_ECI                  [3 x N]                         Acceleration Vector
%                                                       in ECI coordinate
%                                                       frame of reference
%
%
% Outputs:
%---------                                                                %
%r_ECEF                 [3 x N]                         Position Vector in
%                                                       ECEF coordinate
%                                                       frame of reference
%
%v_ECEF                 [3 x N]                         Velocity vector in
%                                                       ECEF coordinate
%                                                       frame of reference
%
%a_ECEF                 [3 x N]                         Acceleration Vector
%                                                       in ECEF coordinate
%                                                       frame of reference
%
% References:
%-------------
%Orbital Mechanics with Numerit, http://www.cdeagle.com/omnum/pdf/csystems.pdf
%
%
% Function Dependencies:
%------------------
% JD2GMST
%------------------------------------------------------------------       %
% Programed by Darin Koblick  07-05-2010                                  %
% Modified on 03/01/2012 to add acceleration vector support               %
%------------------------------------------------------------------       %
function [r_ECEF,v_ECEF,a_ECEF] = ECItoECEF(JD,r_ECI,v_ECI,a_ECI)
%Enforce JD to be [N x 1]
JD = JD(:);

%Calculate the Greenwich Apparent Sideral Time (THETA)
%See http://www.cdeagle.com/omnum/pdf/csystems.pdf equation 27
THETA = JD2GMST(JD);

%Average inertial rotation rate of the earth radians per second
omega_e = 7.29211585275553e-005;

%Assemble the transformation matricies to go from ECI to ECEF
%See http://www.cdeagle.com/omnum/pdf/csystems.pdf equation 26
r_ECEF = squeeze(MultiDimMatrixMultiply(T3D(THETA),r_ECI));
v_ECEF = squeeze(MultiDimMatrixMultiply(T3D(THETA),v_ECI) + ...
    MultiDimMatrixMultiply(Tdot3D(THETA,omega_e),r_ECI));
a_ECEF = squeeze(MultiDimMatrixMultiply(T3D(THETA),a_ECI) + ...
    2.*MultiDimMatrixMultiply(Tdot3D(THETA,omega_e),v_ECI) + ...
    MultiDimMatrixMultiply(Tddot3D(THETA,omega_e),r_ECI));
%----------------------------- End Code-----------------------------------%

function C = MultiDimMatrixMultiply(A,B)
C = sum(bsxfun(@times,A,repmat(permute(B',[3 2 1]),[size(A,2) 1 1])),2);

function T = T3D(THETA)
T = zeros([3 3 length(THETA)]);
T(1,1,:) = cosd(THETA);
T(1,2,:) = sind(THETA);
T(2,1,:) = -T(1,2,:);
T(2,2,:) = T(1,1,:);
T(3,3,:) = ones(size(THETA));

function Tdot = Tdot3D(THETA,omega_e)
Tdot = zeros([3 3 length(THETA)]);
Tdot(1,1,:) = -omega_e.*sind(THETA);
Tdot(1,2,:) = omega_e.*cosd(THETA);
Tdot(2,1,:) = -Tdot(1,2,:);
Tdot(2,2,:) = Tdot(1,1,:);

function Tddot = Tddot3D(THETA,omega_e)
Tddot = zeros([3 3 length(THETA)]);
Tddot(1,1,:) = -(omega_e.^2).*cosd(THETA);
Tddot(1,2,:) = -(omega_e.^2).*sind(THETA);
Tddot(2,1,:) = -Tddot(1,2,:);
Tddot(2,2,:) =  Tddot(1,1,:);

function GMST = JD2GMST(JD)
%Find the Julian Date of the previous midnight, JD0
JD0 = NaN(size(JD));
JDmin = floor(JD)-.5;
JDmax = floor(JD)+.5;
JD0(JD > JDmin) = JDmin(JD > JDmin);
JD0(JD > JDmax) = JDmax(JD > JDmax);
H = (JD-JD0).*24;       %Time in hours past previous midnight
D = JD - 2451545.0;     %Compute the number of days since J2000
D0 = JD0 - 2451545.0;   %Compute the number of days since J2000
T = D./36525;           %Compute the number of centuries since J2000
%Calculate GMST in hours (0h to 24h) ... then convert to degrees
GMST = mod(6.697374558 + 0.06570982441908.*D0  + 1.00273790935.*H + ...
    0.000026.*(T.^2),24).*15;
